simulink model "DD20220329d"  (R2021a)
settings: Solver=VariableStepAuto  StartTime=0.0  StopTime=100  RelTol=1e-3
settings Model: Creator=jaewan  LastModifiedBy=jaewan

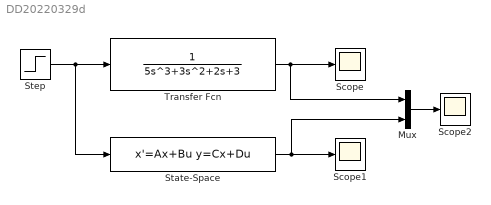
== system DD20220329d ==
  Mux : Mux  Inputs=2
  Scope : Scope
  Scope1 : Scope
  Scope2 : Scope
  State-Space : StateSpace  A=[0 1 0; 0 0 1; -3/5 -2/5 -3/5]  B=[0;0;1/5]  C=[1 0 0]  D=[0]  InitialCondition=0
  Step : Step  After=10  SampleTime=0
  Transfer Fcn : TransferFcn  Denominator=[5 3 2 3]
  wires:
  Step/1 -> State-Space/1, Transfer Fcn/1
  Transfer Fcn/1 -> Mux/1, Scope/1
  State-Space/1 -> Scope1/1, Mux/2
  Mux/1 -> Scope2/1
